simulink model "sas"  (Simulink 6.5)
settings: Solver=ode45  StartTime=0.0  StopTime=10.0  RelTol=1e-3
libraries: cdsFilt x97, cdsMatrix x7, simulink x5, dac x1, cdsParameters x1
(part 1 of 5)
settings Model: Creator=jay  LastModifiedBy=jay
settings DebuggingCC: MultiTaskDSMMsg=warning  MultiTaskCondExecSysMsg=none
settings RTWCC: IncludeERTFirstTime=on

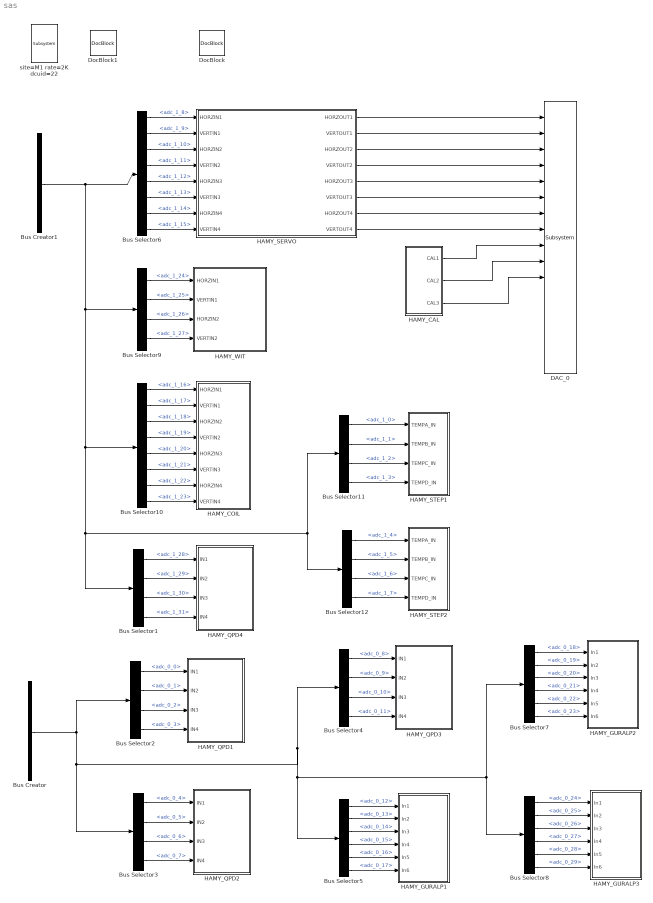
== system sas ==
  Bus Creator : BusCreator  Tag=adc_0  Description=|  Inputs='adc_0_0','adc_0_1','adc_0_2','adc_0_3','adc_0_4','adc_0_5','adc_0_6','adc_0_7','adc_0_8','adc_0_9','adc_0_10','adc_0_11','adc_0_12','adc_0_13','adc_0_14','adc_0_15','adc_0_16','adc_0_17','adc_0_18','adc_0_19','adc_0_20','adc_0_21','adc_0_22','adc_0_23','adc_0_24','adc_0_25','adc_0_26','adc_0_27','adc_0_28','adc_0_29','adc_0_30','adc_0_31'
      | PCI66-16AI64SSA
      | 40Vp-p, 16-bit, 610uV/count
      settings: AttributesFormatString=%<Description>\n%<Tag>
  Bus Creator1 : BusCreator  Tag=adc_1  Description=|  Inputs='adc_1_0','adc_1_1','adc_1_2','adc_1_3','adc_1_4','adc_1_5','adc_1_6','adc_1_7','adc_1_8','adc_1_9','adc_1_10','adc_1_11','adc_1_12','adc_1_13','adc_1_14','adc_1_15','adc_1_16','adc_1_17','adc_1_18','adc_1_19','adc_1_20','adc_1_21','adc_1_22','adc_1_23','adc_1_24','adc_1_25','adc_1_26','adc_1_27','adc_1_28','adc_1_29','adc_1_30','adc_1_31'
      | PCI66-16AI64SSA
      | 40Vp-p, 16-bit, 610uV/count
      settings: AttributesFormatString=%<Description>\n%<Tag>
  Bus Selector1 : BusSelector  Description=ADC Selector  OutputSignals=adc_1_28,adc_1_29,adc_1_30,adc_1_31
      settings: AttributesFormatString=%<Description>
  Bus Selector10 : BusSelector  Description=ADC Selector  OutputSignals=adc_1_16,adc_1_17,adc_1_18,adc_1_19,adc_1_20,adc_1_21,adc_1_22,adc_1_23
      settings: AttributesFormatString=%<Description>
  Bus Selector11 : BusSelector  Description=ADC Selector  OutputSignals=adc_1_0,adc_1_1,adc_1_2,adc_1_3
      settings: AttributesFormatString=%<Description>
  Bus Selector12 : BusSelector  Description=ADC Selector  OutputSignals=adc_1_4,adc_1_5,adc_1_6,adc_1_7
      settings: AttributesFormatString=%<Description>
  Bus Selector2 : BusSelector  Description=ADC Selector  OutputSignals=adc_0_0,adc_0_1,adc_0_2,adc_0_3
      settings: AttributesFormatString=%<Description>
  Bus Selector3 : BusSelector  Description=ADC Selector  OutputSignals=adc_0_4,adc_0_5,adc_0_6,adc_0_7
      settings: AttributesFormatString=%<Description>
  Bus Selector4 : BusSelector  Description=ADC Selector  OutputSignals=adc_0_8,adc_0_9,adc_0_10,adc_0_11
      settings: AttributesFormatString=%<Description>
  Bus Selector5 : BusSelector  Description=ADC Selector  OutputSignals=adc_0_12,adc_0_13,adc_0_14,adc_0_15,adc_0_16,adc_0_17
      settings: AttributesFormatString=%<Description>
  Bus Selector6 : BusSelector  Description=ADC Selector  OutputSignals=adc_1_8,adc_1_9,adc_1_10,adc_1_11,adc_1_12,adc_1_13,adc_1_14,adc_1_15
      settings: AttributesFormatString=%<Description>
  Bus Selector7 : BusSelector  Description=ADC Selector  OutputSignals=adc_0_18,adc_0_19,adc_0_20,adc_0_21,adc_0_22,adc_0_23
      settings: AttributesFormatString=%<Description>
  Bus Selector8 : BusSelector  Description=ADC Selector  OutputSignals=adc_0_24,adc_0_25,adc_0_26,adc_0_27,adc_0_28,adc_0_29
      settings: AttributesFormatString=%<Description>
  Bus Selector9 : BusSelector  Description=ADC Selector  OutputSignals=adc_1_24,adc_1_25,adc_1_26,adc_1_27
      settings: AttributesFormatString=%<Description>
  DAC_0 : dac/Subsystem  Description=|  SystemSampleTime=-1
      | PCI66-16AO16
      | 20Vp-p, 16-bit, 305uV/count
      settings: AttributesFormatString=%<Description>
  DocBlock : simulink/Model-Wide Utilities/DocBlock  Tag=HAM SAS System Overview  SystemSampleTime=-1  DocumentType=Text
      settings: AttributesFormatString=%<Tag>
  DocBlock1 : simulink/Model-Wide Utilities/DocBlock  Tag=SW Install  SystemSampleTime=-1  DocumentType=Text
      settings: AttributesFormatString=%<Tag>
  HAMY_CAL : Subsystem  Description=Guralp Calibration Signals
      settings: AttributesFormatString=%<Description>
  HAMY_COIL : Subsystem  Description=Actuator Coil Voltage Monitors
      settings: AttributesFormatString=%<Description>
  HAMY_GURALP1 : Subsystem  Description=|
      | Guralp Monitors- VeVERT, VeN/S, VeE/W,
      | MassVert, MassN/S, MassE/W
      settings: AttributesFormatString=%<Description>
  HAMY_GURALP2 : Subsystem  Description=|
      | Guralp Monitors- VeVERT, VeN/S, VeE/W,
      | MassVert, MassN/S, MassE/W
      settings: AttributesFormatString=%<Description>
  HAMY_GURALP3 : Subsystem  Description=|
      | Guralp Monitors- VeVERT, VeN/S, VeE/W,
      | MassVert, MassN/S, MassE/W
      settings: AttributesFormatString=%<Description>
  HAMY_QPD1 : Subsystem  Description=QPD Monitors of Table-- SUM, PIT, YAW
      settings: AttributesFormatString=%<Description>
  HAMY_QPD2 : Subsystem  Description=QPD Monitors of Table-- SUM, PIT, YAW
      settings: AttributesFormatString=%<Description>
  HAMY_QPD3 : Subsystem  Description=QPD Monitors of Table-- SUM, PIT, YAW
      settings: AttributesFormatString=%<Description>
  HAMY_QPD4 : Subsystem  Description=QPD Monitors of Table-- SUM, PIT, YAW
      settings: AttributesFormatString=%<Description>
  HAMY_SERVO : Subsystem  Description=Servo-- LVDT Sensor Signal to DOF to Actuator Outputs
      settings: AttributesFormatString=%<Description>
  HAMY_STEP1 : Subsystem  Description=Stepper Motor Temps
      settings: AttributesFormatString=%<Description>
  HAMY_STEP2 : Subsystem  Description=Stepper Motor Temps
      settings: AttributesFormatString=%<Description>
  HAMY_WIT : Subsystem  Description=Witness LVDT Sensor Signals
      settings: AttributesFormatString=%<Description>
  site=M1 rate=2K dcuid=22 : cdsParameters/Subsystem  Tag=cdsParameters  SystemSampleTime=-1
      settings: AttributesFormatString=%<Tag>
  wires:
  Bus Creator1/1 -> Bus Selector6/1, Bus Selector10/1, Bus Selector1/1, Bus Selector11/1, Bus Selector12/1, Bus Selector9/1
  Bus Selector6/1 -> HAMY_SERVO/1(HORZIN1)  "<adc_1_8>"
  Bus Selector6/2 -> HAMY_SERVO/2(VERTIN1)  "<adc_1_9>"
  Bus Selector6/3 -> HAMY_SERVO/3(HORZIN2)  "<adc_1_10>"
  Bus Selector6/4 -> HAMY_SERVO/4(VERTIN2)  "<adc_1_11>"
  Bus Selector6/5 -> HAMY_SERVO/5(HORZIN3)  "<adc_1_12>"
  Bus Selector6/6 -> HAMY_SERVO/6(VERTIN3)  "<adc_1_13>"
  Bus Selector6/7 -> HAMY_SERVO/7(HORZIN4)  "<adc_1_14>"
  Bus Selector6/8 -> HAMY_SERVO/8(VERTIN4)  "<adc_1_15>"
  HAMY_CAL/1(CAL1) -> DAC_0/9
  HAMY_CAL/2(CAL2) -> DAC_0/10
  HAMY_CAL/3(CAL3) -> DAC_0/11
  Bus Selector1/1 -> HAMY_QPD4/1(IN1)  "<adc_1_28>"
  Bus Selector1/2 -> HAMY_QPD4/2(IN2)  "<adc_1_29>"
  Bus Selector1/3 -> HAMY_QPD4/3(IN3)  "<adc_1_30>"
  Bus Selector1/4 -> HAMY_QPD4/4(IN4)  "<adc_1_31>"
  Bus Creator/1 -> Bus Selector2/1, Bus Selector3/1, Bus Selector4/1, Bus Selector5/1, Bus Selector8/1, Bus Selector7/1
  Bus Selector2/1 -> HAMY_QPD1/1(IN1)  "<adc_0_0>"
  Bus Selector2/2 -> HAMY_QPD1/2(IN2)  "<adc_0_1>"
  Bus Selector2/3 -> HAMY_QPD1/3(IN3)  "<adc_0_2>"
  Bus Selector2/4 -> HAMY_QPD1/4(IN4)  "<adc_0_3>"
  Bus Selector3/1 -> HAMY_QPD2/1(IN1)  "<adc_0_4>"
  Bus Selector3/2 -> HAMY_QPD2/2(IN2)  "<adc_0_5>"
  Bus Selector3/3 -> HAMY_QPD2/3(IN3)  "<adc_0_6>"
  Bus Selector3/4 -> HAMY_QPD2/4(IN4)  "<adc_0_7>"
  Bus Selector4/1 -> HAMY_QPD3/1(IN1)  "<adc_0_8>"
  Bus Selector4/2 -> HAMY_QPD3/2(IN2)  "<adc_0_9>"
  Bus Selector4/3 -> HAMY_QPD3/3(IN3)  "<adc_0_10>"
  Bus Selector4/4 -> HAMY_QPD3/4(IN4)  "<adc_0_11>"
  Bus Selector5/1 -> HAMY_GURALP1/1(In1)  "<adc_0_12>"
  Bus Selector5/2 -> HAMY_GURALP1/2(In2)  "<adc_0_13>"
  Bus Selector5/3 -> HAMY_GURALP1/3(In3)  "<adc_0_14>"
  Bus Selector5/4 -> HAMY_GURALP1/4(In4)  "<adc_0_15>"
  Bus Selector5/5 -> HAMY_GURALP1/5(In5)  "<adc_0_16>"
  Bus Selector5/6 -> HAMY_GURALP1/6(In6)  "<adc_0_17>"
  Bus Selector7/1 -> HAMY_GURALP2/1(In1)  "<adc_0_18>"
  Bus Selector7/2 -> HAMY_GURALP2/2(In2)  "<adc_0_19>"
  Bus Selector7/3 -> HAMY_GURALP2/3(In3)  "<adc_0_20>"
  Bus Selector7/4 -> HAMY_GURALP2/4(In4)  "<adc_0_21>"
  Bus Selector7/5 -> HAMY_GURALP2/5(In5)  "<adc_0_22>"
  Bus Selector7/6 -> HAMY_GURALP2/6(In6)  "<adc_0_23>"
  Bus Selector8/1 -> HAMY_GURALP3/1(In1)  "<adc_0_24>"
  Bus Selector8/2 -> HAMY_GURALP3/2(In2)  "<adc_0_25>"
  Bus Selector8/3 -> HAMY_GURALP3/3(In3)  "<adc_0_26>"
  Bus Selector8/4 -> HAMY_GURALP3/4(In4)  "<adc_0_27>"
  Bus Selector8/5 -> HAMY_GURALP3/5(In5)  "<adc_0_28>"
  Bus Selector8/6 -> HAMY_GURALP3/6(In6)  "<adc_0_29>"
  Bus Selector10/1 -> HAMY_COIL/1(HORZIN1)  "<adc_1_16>"
  Bus Selector10/2 -> HAMY_COIL/2(VERTIN1)  "<adc_1_17>"
  Bus Selector10/3 -> HAMY_COIL/3(HORZIN2)  "<adc_1_18>"
  Bus Selector10/4 -> HAMY_COIL/4(VERTIN2)  "<adc_1_19>"
  Bus Selector10/5 -> HAMY_COIL/5(HORZIN3)  "<adc_1_20>"
  Bus Selector10/6 -> HAMY_COIL/6(VERTIN3)  "<adc_1_21>"
  Bus Selector10/7 -> HAMY_COIL/7(HORZIN4)  "<adc_1_22>"
  Bus Selector10/8 -> HAMY_COIL/8(VERTIN4)  "<adc_1_23>"
  Bus Selector11/1 -> HAMY_STEP1/1(TEMPA_IN)  "<adc_1_0>"
  Bus Selector11/2 -> HAMY_STEP1/2(TEMPB_IN)  "<adc_1_1>"
  Bus Selector11/3 -> HAMY_STEP1/3(TEMPC_IN)  "<adc_1_2>"
  Bus Selector11/4 -> HAMY_STEP1/4(TEMPD_IN)  "<adc_1_3>"
  Bus Selector12/1 -> HAMY_STEP2/1(TEMPA_IN)  "<adc_1_4>"
  Bus Selector12/2 -> HAMY_STEP2/2(TEMPB_IN)  "<adc_1_5>"
  Bus Selector12/3 -> HAMY_STEP2/3(TEMPC_IN)  "<adc_1_6>"
  Bus Selector12/4 -> HAMY_STEP2/4(TEMPD_IN)  "<adc_1_7>"
  Bus Selector9/1 -> HAMY_WIT/1(HORZIN1)  "<adc_1_24>"
  Bus Selector9/2 -> HAMY_WIT/2(VERTIN1)  "<adc_1_25>"
  Bus Selector9/3 -> HAMY_WIT/3(HORZIN2)  "<adc_1_26>"
  Bus Selector9/4 -> HAMY_WIT/4(VERTIN2)  "<adc_1_27>"
  HAMY_SERVO/1(HORZOUT1) -> DAC_0/1
  HAMY_SERVO/2(VERTOUT1) -> DAC_0/2
  HAMY_SERVO/3(HORZOUT2) -> DAC_0/3
  HAMY_SERVO/4(VERTOUT2) -> DAC_0/4
  HAMY_SERVO/5(HORZOUT3) -> DAC_0/5
  HAMY_SERVO/6(VERTOUT3) -> DAC_0/6
  HAMY_SERVO/7(HORZOUT4) -> DAC_0/7
  HAMY_SERVO/8(VERTOUT4) -> DAC_0/8

== system sas/HAMY_CAL ==
  DocBlock : simulink/Model-Wide Utilities/DocBlock  Tag=Guralp Calibration Overview  SystemSampleTime=-1  DocumentType=Text
      settings: AttributesFormatString=%<Tag>
  GARULP1 : cdsFilt/Subsystem  Tag=cdsFilt  Description=|  SystemSampleTime=-1
      | Purpose:                                                                                                                                                                                                                                  
      | Standard CDS IIR filter module.                                                                                                                                                                                                           
      |                                                                                                                                                                                                                                           
      | Operation:                                                                                                                                                                                                                                
      | Consists of 10 second order section IIR filters, plus a ramped gain stage. In FE code, also provides pre-defined test points and excitation channel inputs. The filter coefficients are defined in the LIGO system using the 'foton' tool.
      |                                                                                                                                                                                                                                           
      | Usage:                                                                                                                                                                                                                                    
      | Name the part with the desired filter module name.
      settings: AttributesFormatString=%<Tag>
  GARULP2 : cdsFilt/Subsystem  Tag=cdsFilt  Description=|  SystemSampleTime=-1
      | Purpose:                                                                                                                                                                                                                                  
      | Standard CDS IIR filter module.                                                                                                                                                                                                           
      |                                                                                                                                                                                                                                           
      | Operation:                                                                                                                                                                                                                                
      | Consists of 10 second order section IIR filters, plus a ramped gain stage. In FE code, also provides pre-defined test points and excitation channel inputs. The filter coefficients are defined in the LIGO system using the 'foton' tool.
      |                                                                                                                                                                                                                                           
      | Usage:                                                                                                                                                                                                                                    
      | Name the part with the desired filter module name.
      settings: AttributesFormatString=%<Tag>
  GARULP3 : cdsFilt/Subsystem  Tag=cdsFilt  Description=|  SystemSampleTime=-1
      | Purpose:                                                                                                                                                                                                                                  
      | Standard CDS IIR filter module.                                                                                                                                                                                                           
      |                                                                                                                                                                                                                                           
      | Operation:                                                                                                                                                                                                                                
      | Consists of 10 second order section IIR filters, plus a ramped gain stage. In FE code, also provides pre-defined test points and excitation channel inputs. The filter coefficients are defined in the LIGO system using the 'foton' tool.
      |                                                                                                                                                                                                                                           
      | Usage:                                                                                                                                                                                                                                    
      | Name the part with the desired filter module name.
      settings: AttributesFormatString=%<Tag>
  Ground : Ground
  Ground1 : Ground
  Ground2 : Ground
  CAL1 : Outport
  CAL2 : Outport  Port=2
  CAL3 : Outport  Port=3
  wires:
  GARULP1/1 -> CAL1/1
  Ground1/1 -> GARULP2/1
  GARULP2/1 -> CAL2/1
  Ground2/1 -> GARULP3/1
  GARULP3/1 -> CAL3/1
  Ground/1 -> GARULP1/1

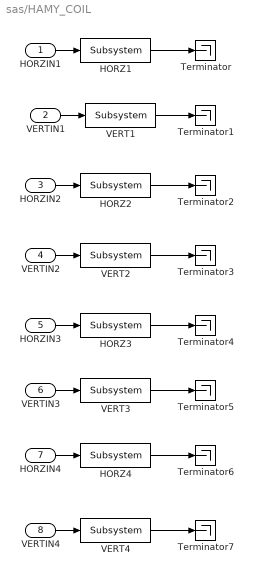
== system sas/HAMY_COIL ==
  HORZIN1 : Inport
  VERTIN1 : Inport  Port=2
  HORZIN2 : Inport  Port=3
  VERTIN2 : Inport  Port=4
  HORZIN3 : Inport  Port=5
  VERTIN3 : Inport  Port=6
  HORZIN4 : Inport  Port=7
  VERTIN4 : Inport  Port=8
  HORZ1 : cdsFilt/Subsystem  Tag=cdsFilt  Description=|  SystemSampleTime=-1
      | Purpose:                                                                                                                                                                                                                                  
      | Standard CDS IIR filter module.                                                                                                                                                                                                           
      |                                                                                                                                                                                                                                           
      | Operation:                                                                                                                                                                                                                                
      | Consists of 10 second order section IIR filters, plus a ramped gain stage. In FE code, also provides pre-defined test points and excitation channel inputs. The filter coefficients are defined in the LIGO system using the 'foton' tool.
      |                                                                                                                                                                                                                                           
      | Usage:                                                                                                                                                                                                                                    
      | Name the part with the desired filter module name.
      settings: AttributesFormatString=%<Tag>
  HORZ2 : cdsFilt/Subsystem  Tag=cdsFilt  Description=|  SystemSampleTime=-1
      | Purpose:                                                                                                                                                                                                                                  
      | Standard CDS IIR filter module.                                                                                                                                                                                                           
      |                                                                                                                                                                                                                                           
      | Operation:                                                                                                                                                                                                                                
      | Consists of 10 second order section IIR filters, plus a ramped gain stage. In FE code, also provides pre-defined test points and excitation channel inputs. The filter coefficients are defined in the LIGO system using the 'foton' tool.
      |                                                                                                                                                                                                                                           
      | Usage:                                                                                                                                                                                                                                    
      | Name the part with the desired filter module name.
      settings: AttributesFormatString=%<Tag>
  HORZ3 : cdsFilt/Subsystem  Tag=cdsFilt  Description=|  SystemSampleTime=-1
      | Purpose:                                                                                                                                                                                                                                  
      | Standard CDS IIR filter module.                                                                                                                                                                                                           
      |                                                                                                                                                                                                                                           
      | Operation:                                                                                                                                                                                                                                
      | Consists of 10 second order section IIR filters, plus a ramped gain stage. In FE code, also provides pre-defined test points and excitation channel inputs. The filter coefficients are defined in the LIGO system using the 'foton' tool.
      |                                                                                                                                                                                                                                           
      | Usage:                                                                                                                                                                                                                                    
      | Name the part with the desired filter module name.
      settings: AttributesFormatString=%<Tag>
  HORZ4 : cdsFilt/Subsystem  Tag=cdsFilt  Description=|  SystemSampleTime=-1
      | Purpose:                                                                                                                                                                                                                                  
      | Standard CDS IIR filter module.                                                                                                                                                                                                           
      |                                                                                                                                                                                                                                           
      | Operation:                                                                                                                                                                                                                                
      | Consists of 10 second order section IIR filters, plus a ramped gain stage. In FE code, also provides pre-defined test points and excitation channel inputs. The filter coefficients are defined in the LIGO system using the 'foton' tool.
      |                                                                                                                                                                                                                                           
      | Usage:                                                                                                                                                                                                                                    
      | Name the part with the desired filter module name.
      settings: AttributesFormatString=%<Tag>
  Terminator{,1..7} (8 alike) : Terminator
  VERT1 : cdsFilt/Subsystem  Tag=cdsFilt  Description=|  SystemSampleTime=-1
      | Purpose:                                                                                                                                                                                                                                  
      | Standard CDS IIR filter module.                                                                                                                                                                                                           
      |                                                                                                                                                                                                                                           
      | Operation:                                                                                                                                                                                                                                
      | Consists of 10 second order section IIR filters, plus a ramped gain stage. In FE code, also provides pre-defined test points and excitation channel inputs. The filter coefficients are defined in the LIGO system using the 'foton' tool.
      |                                                                                                                                                                                                                                           
      | Usage:                                                                                                                                                                                                                                    
      | Name the part with the desired filter module name.
      settings: AttributesFormatString=%<Tag>
  VERT2 : cdsFilt/Subsystem  Tag=cdsFilt  Description=|  SystemSampleTime=-1
      | Purpose:                                                                                                                                                                                                                                  
      | Standard CDS IIR filter module.                                                                                                                                                                                                           
      |                                                                                                                                                                                                                                           
      | Operation:                                                                                                                                                                                                                                
      | Consists of 10 second order section IIR filters, plus a ramped gain stage. In FE code, also provides pre-defined test points and excitation channel inputs. The filter coefficients are defined in the LIGO system using the 'foton' tool.
      |                                                                                                                                                                                                                                           
      | Usage:                                                                                                                                                                                                                                    
      | Name the part with the desired filter module name.
      settings: AttributesFormatString=%<Tag>
  VERT3 : cdsFilt/Subsystem  Tag=cdsFilt  Description=|  SystemSampleTime=-1
      | Purpose:                                                                                                                                                                                                                                  
      | Standard CDS IIR filter module.                                                                                                                                                                                                           
      |                                                                                                                                                                                                                                           
      | Operation:                                                                                                                                                                                                                                
      | Consists of 10 second order section IIR filters, plus a ramped gain stage. In FE code, also provides pre-defined test points and excitation channel inputs. The filter coefficients are defined in the LIGO system using the 'foton' tool.
      |                                                                                                                                                                                                                                           
      | Usage:                                                                                                                                                                                                                                    
      | Name the part with the desired filter module name.
      settings: AttributesFormatString=%<Tag>
  VERT4 : cdsFilt/Subsystem  Tag=cdsFilt  Description=|  SystemSampleTime=-1
      | Purpose:                                                                                                                                                                                                                                  
      | Standard CDS IIR filter module.                                                                                                                                                                                                           
      |                                                                                                                                                                                                                                           
      | Operation:                                                                                                                                                                                                                                
      | Consists of 10 second order section IIR filters, plus a ramped gain stage. In FE code, also provides pre-defined test points and excitation channel inputs. The filter coefficients are defined in the LIGO system using the 'foton' tool.
      |                                                                                                                                                                                                                                           
      | Usage:                                                                                                                                                                                                                                    
      | Name the part with the desired filter module name.
      settings: AttributesFormatString=%<Tag>
  wires:
  HORZIN1/1 -> HORZ1/1
  HORZ1/1 -> Terminator/1
  VERTIN1/1 -> VERT1/1
  VERT1/1 -> Terminator1/1
  HORZIN2/1 -> HORZ2/1
  HORZ2/1 -> Terminator2/1
  VERTIN2/1 -> VERT2/1
  VERT2/1 -> Terminator3/1
  HORZIN3/1 -> HORZ3/1
  HORZ3/1 -> Terminator4/1
  VERTIN3/1 -> VERT3/1
  VERT3/1 -> Terminator5/1
  HORZIN4/1 -> HORZ4/1
  HORZ4/1 -> Terminator6/1
  VERTIN4/1 -> VERT4/1
  VERT4/1 -> Terminator7/1

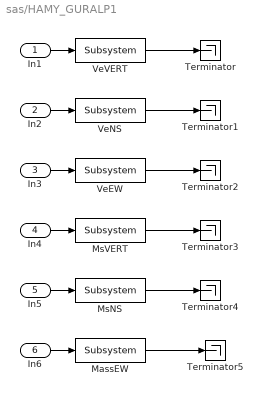
== system sas/HAMY_GURALP1 ==
  In1 : Inport
  In2 : Inport  Port=2
  In3 : Inport  Port=3
  In4 : Inport  Port=4
  In5 : Inport  Port=5
  In6 : Inport  Port=6
  MassEW : cdsFilt/Subsystem  Tag=cdsFilt  Description=|  SystemSampleTime=-1
      | Purpose:                                                                                                                                                                                                                                  
      | Standard CDS IIR filter module.                                                                                                                                                                                                           
      |                                                                                                                                                                                                                                           
      | Operation:                                                                                                                                                                                                                                
      | Consists of 10 second order section IIR filters, plus a ramped gain stage. In FE code, also provides pre-defined test points and excitation channel inputs. The filter coefficients are defined in the LIGO system using the 'foton' tool.
      |                                                                                                                                                                                                                                           
      | Usage:                                                                                                                                                                                                                                    
      | Name the part with the desired filter module name.
      settings: AttributesFormatString=%<Tag>
  MsNS : cdsFilt/Subsystem  Tag=cdsFilt  Description=|  SystemSampleTime=-1
      | Purpose:                                                                                                                                                                                                                                  
      | Standard CDS IIR filter module.                                                                                                                                                                                                           
      |                                                                                                                                                                                                                                           
      | Operation:                                                                                                                                                                                                                                
      | Consists of 10 second order section IIR filters, plus a ramped gain stage. In FE code, also provides pre-defined test points and excitation channel inputs. The filter coefficients are defined in the LIGO system using the 'foton' tool.
      |                                                                                                                                                                                                                                           
      | Usage:                                                                                                                                                                                                                                    
      | Name the part with the desired filter module name.
      settings: AttributesFormatString=%<Tag>
  MsVERT : cdsFilt/Subsystem  Tag=cdsFilt  Description=|  SystemSampleTime=-1
      | Purpose:                                                                                                                                                                                                                                  
      | Standard CDS IIR filter module.                                                                                                                                                                                                           
      |                                                                                                                                                                                                                                           
      | Operation:                                                                                                                                                                                                                                
      | Consists of 10 second order section IIR filters, plus a ramped gain stage. In FE code, also provides pre-defined test points and excitation channel inputs. The filter coefficients are defined in the LIGO system using the 'foton' tool.
      |                                                                                                                                                                                                                                           
      | Usage:                                                                                                                                                                                                                                    
      | Name the part with the desired filter module name.
      settings: AttributesFormatString=%<Tag>
  Terminator{,1..5} (6 alike) : Terminator
  VeEW : cdsFilt/Subsystem  Tag=cdsFilt  Description=|  SystemSampleTime=-1
      | Purpose:                                                                                                                                                                                                                                  
      | Standard CDS IIR filter module.                                                                                                                                                                                                           
      |                                                                                                                                                                                                                                           
      | Operation:                                                                                                                                                                                                                                
      | Consists of 10 second order section IIR filters, plus a ramped gain stage. In FE code, also provides pre-defined test points and excitation channel inputs. The filter coefficients are defined in the LIGO system using the 'foton' tool.
      |                                                                                                                                                                                                                                           
      | Usage:                                                                                                                                                                                                                                    
      | Name the part with the desired filter module name.
      settings: AttributesFormatString=%<Tag>
  VeNS : cdsFilt/Subsystem  Tag=cdsFilt  Description=|  SystemSampleTime=-1
      | Purpose:                                                                                                                                                                                                                                  
      | Standard CDS IIR filter module.                                                                                                                                                                                                           
      |                                                                                                                                                                                                                                           
      | Operation:                                                                                                                                                                                                                                
      | Consists of 10 second order section IIR filters, plus a ramped gain stage. In FE code, also provides pre-defined test points and excitation channel inputs. The filter coefficients are defined in the LIGO system using the 'foton' tool.
      |                                                                                                                                                                                                                                           
      | Usage:                                                                                                                                                                                                                                    
      | Name the part with the desired filter module name.
      settings: AttributesFormatString=%<Tag>
  VeVERT : cdsFilt/Subsystem  Tag=cdsFilt  Description=|  SystemSampleTime=-1
      | Purpose:                                                                                                                                                                                                                                  
      | Standard CDS IIR filter module.                                                                                                                                                                                                           
      |                                                                                                                                                                                                                                           
      | Operation:                                                                                                                                                                                                                                
      | Consists of 10 second order section IIR filters, plus a ramped gain stage. In FE code, also provides pre-defined test points and excitation channel inputs. The filter coefficients are defined in the LIGO system using the 'foton' tool.
      |                                                                                                                                                                                                                                           
      | Usage:                                                                                                                                                                                                                                    
      | Name the part with the desired filter module name.
      settings: AttributesFormatString=%<Tag>
  wires:
  In1/1 -> VeVERT/1
  VeVERT/1 -> Terminator/1
  In2/1 -> VeNS/1
  VeNS/1 -> Terminator1/1
  In3/1 -> VeEW/1
  VeEW/1 -> Terminator2/1
  In4/1 -> MsVERT/1
  MsVERT/1 -> Terminator3/1
  In5/1 -> MsNS/1
  MsNS/1 -> Terminator4/1
  In6/1 -> MassEW/1
  MassEW/1 -> Terminator5/1
